simulink model "digital_filter"  (R2018b)
settings: Solver=ode4  StartTime=0.0  StopTime=0.08  FixedStep=5e-6  RelTol=1e-3
undefined symbols (not defined in the file or in its folder): DiscIntNeverNeededParam
libraries: powerlib_meascontrol x8, dsparch4 x1
settings Model: Creator=Alexey  LastModifiedBy=Alexey

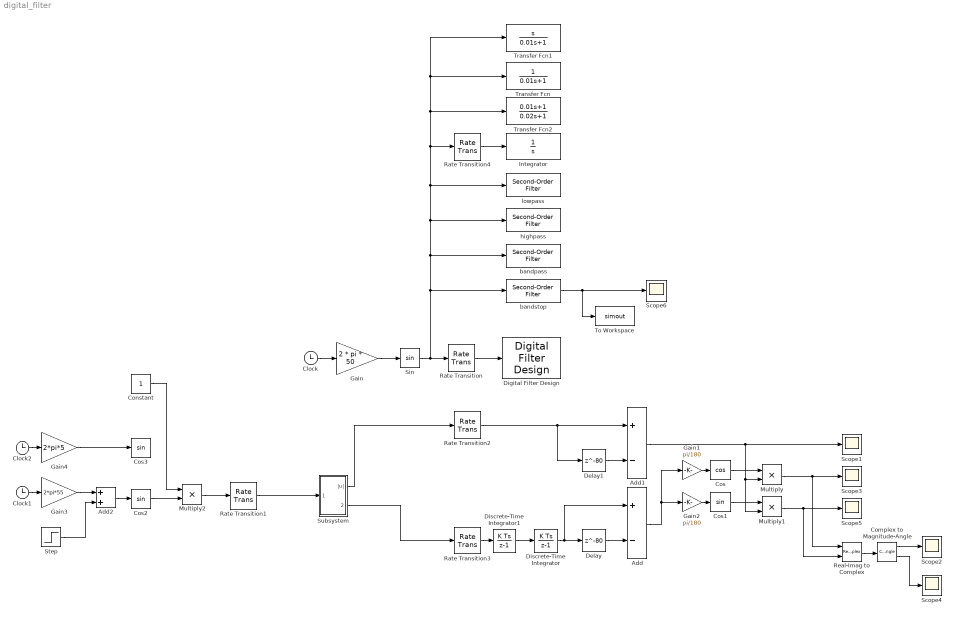
== system digital_filter ==
  Add : Sum  Inputs=+-
  Add1 : Sum  Inputs=+-
  Add2 : Sum
  Clock : Clock
  Clock1 : Clock
  Clock2 : Clock
  Complex to Magnitude-Angle : ComplexToMagnitudeAngle
  Constant : Constant
  Cos : Trigonometry  Operator=cos
  Cos1 : Trigonometry
  Cos2 : Trigonometry
  Cos3 : Trigonometry
  Delay : Delay  DelayLength=80
  Delay1 : Delay  DelayLength=80
  Digital Filter Design : dsparch4/Digital Filter Design  mwdsp_browser_bugfix_var=off
  Discrete-Time Integrator : DiscreteIntegrator  SampleTime=-1  ICPrevOutput=DiscIntNeverNeededParam  ICPrevScaledInput=DiscIntNeverNeededParam
  Discrete-Time Integrator1 : DiscreteIntegrator  SampleTime=-1  ICPrevOutput=DiscIntNeverNeededParam  ICPrevScaledInput=DiscIntNeverNeededParam
  Gain : Gain  Gain=2 * pi * 50
  Gain1 : Gain  Gain=pi/180
  Gain2 : Gain  Gain=pi/180
  Gain3 : Gain  Gain=2*pi*55
  Gain4 : Gain  Gain=2*pi*5
  Integrator : Integrator
  Multiply : Product
  Multiply1 : Product
  Multiply2 : Product
  Rate Transition : RateTransition  Integrity=off  Deterministic=off  OutPortSampleTime=1 / 4000
  Rate Transition1 : RateTransition  Integrity=off  Deterministic=off  OutPortSampleTime=1/4000
  Rate Transition2 : RateTransition  Integrity=off  Deterministic=off  OutPortSampleTime=1/4000
  Rate Transition3 : RateTransition  Integrity=off  Deterministic=off  OutPortSampleTime=1/4000
  Rate Transition4 : RateTransition  Integrity=off  Deterministic=off  OutPortSampleTime=1 / 4000
  Real-Imag to Complex : RealImagToComplex
  Scope{1..6} (6 alike) : Scope
  Sin : Trigonometry
  Step : Step  Time=0.5  After=30*pi/180  SampleTime=0
  Subsystem : Subsystem
  To Workspace : ToWorkspace  VariableName=simout  SampleTime=1/4000
  Transfer Fcn : TransferFcn  Numerator=[0 1]  Denominator=[0.01 1]
  Transfer Fcn1 : TransferFcn  Numerator=[1 0]  Denominator=[0.01 1]
  Transfer Fcn2 : TransferFcn  Numerator=[0.01 1]  Denominator=[0.02 1]
  bandpass : powerlib_meascontrol/Filters/Second-Order Filter  FilterType=Bandpass  Fo=120  Zeta=0.707  Ts=0  Initialize=off  Vac_Init="[0,  0,  60]"  Vdc_Init=0  PlotResponse=off  FreqRange=[0, 500, 1]
      settings: SourceProductName=Simscape Power Systems  SourceProductBaseCode=PS
  bandstop : powerlib_meascontrol/Filters/Second-Order Filter  FilterType=Bandstop (Notch)  Fo=120  Zeta=0.707  Ts=0  Initialize=off  Vac_Init="[0,  0,  60]"  Vdc_Init=0  PlotResponse=off  FreqRange=[0, 500, 1]
      settings: SourceProductName=Simscape Power Systems  SourceProductBaseCode=PS
  highpass : powerlib_meascontrol/Filters/Second-Order Filter  FilterType=Highpass  Fo=120  Zeta=0.707  Ts=0  Initialize=off  Vac_Init="[0,  0,  60]"  Vdc_Init=0  PlotResponse=off  FreqRange=[0, 500, 1]
      settings: SourceProductName=Simscape Power Systems  SourceProductBaseCode=PS
  lowpass : powerlib_meascontrol/Filters/Second-Order Filter  FilterType=Lowpass  Fo=120  Zeta=0.707  Ts=0  Initialize=off  Vac_Init="[0,  0,  60]"  Vdc_Init=0  PlotResponse=off  FreqRange=[0, 500, 1]
      settings: SourceProductName=Simscape Power Systems  SourceProductBaseCode=PS
  wires:
  Clock/1 -> Gain/1
  Gain/1 -> Sin/1
  Sin/1 -> bandstop/1, bandpass/1, lowpass/1, Transfer Fcn2/1, Transfer Fcn1/1, Transfer Fcn/1, Rate Transition4/1, highpass/1, Rate Transition/1
  Rate Transition/1 -> Digital Filter Design/1
  Subsystem/2(arg) -> Rate Transition3/1
  Discrete-Time Integrator/1 -> Add/1, Delay/1
  Delay/1 -> Add/2
  Add/1 -> Gain1/1, Gain2/1
  Delay1/1 -> Add1/2
  Discrete-Time Integrator1/1 -> Discrete-Time Integrator/1
  Rate Transition1/1 -> Subsystem/1(input)
  Subsystem/1(|u|) -> Rate Transition2/1
  Add1/1 -> Multiply1/2, Multiply/2, Scope1/1
  Gain1/1 -> Cos/1
  Gain2/1 -> Cos1/1
  Cos/1 -> Multiply/1
  Cos1/1 -> Multiply1/1
  Multiply/1 -> Real-Imag to Complex/1, Scope3/1
  Multiply1/1 -> Real-Imag to Complex/2, Scope5/1
  Rate Transition2/1 -> Delay1/1, Add1/1
  Rate Transition3/1 -> Discrete-Time Integrator1/1
  Clock1/1 -> Gain3/1
  Gain3/1 -> Add2/1
  Step/1 -> Add2/2
  Add2/1 -> Cos2/1
  Cos2/1 -> Multiply2/2
  Real-Imag to Complex/1 -> Complex to Magnitude-Angle/1
  Complex to Magnitude-Angle/1 -> Scope2/1
  Multiply2/1 -> Rate Transition1/1
  Clock2/1 -> Gain4/1
  Gain4/1 -> Cos3/1
  Complex to Magnitude-Angle/2 -> Scope4/1
  Constant/1 -> Multiply2/1
  bandstop/1 -> To Workspace/1, Scope6/1
  Rate Transition4/1 -> Integrator/1

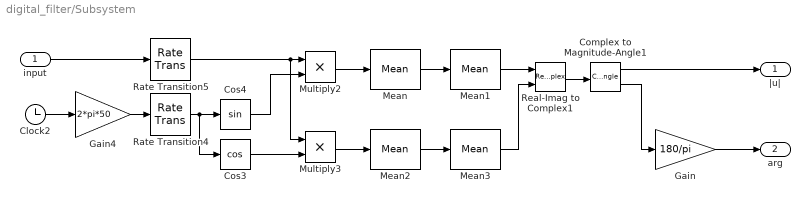
== system digital_filter/Subsystem ==
  input : Inport
  Clock2 : Clock
  Complex to Magnitude-Angle1 : ComplexToMagnitudeAngle
  Cos3 : Trigonometry  Operator=cos
  Cos4 : Trigonometry
  Gain : Gain  Gain=180/pi
  Gain4 : Gain  Gain=2*pi*50
  Mean{,1..3} (4 alike) : powerlib_meascontrol/Measurements/Mean  Freq=50  Vinit=0  Ts=1/4000
  Multiply2 : Product
  Multiply3 : Product
  Rate Transition4 : RateTransition  Integrity=off  Deterministic=off  OutPortSampleTime=1/4000
  Rate Transition5 : RateTransition  Integrity=off  Deterministic=off  OutPortSampleTime=1/4000
  Real-Imag to Complex1 : RealImagToComplex
  |u| : Outport
  arg : Outport  Port=2
  wires:
  Real-Imag to Complex1/1 -> Complex to Magnitude-Angle1/1
  Rate Transition4/1 -> Cos3/1, Cos4/1
  Clock2/1 -> Gain4/1
  Cos3/1 -> Multiply3/2
  Rate Transition5/1 -> Multiply3/1, Multiply2/1
  Multiply2/1 -> Mean/1
  Mean1/1 -> Real-Imag to Complex1/1
  Mean/1 -> Mean1/1
  Gain4/1 -> Rate Transition4/1
  Multiply3/1 -> Mean2/1
  Mean2/1 -> Mean3/1
  Cos4/1 -> Multiply2/2
  Mean3/1 -> Real-Imag to Complex1/2
  Complex to Magnitude-Angle1/1 -> |u|/1
  Complex to Magnitude-Angle1/2 -> Gain/1
  input/1 -> Rate Transition5/1
  Gain/1 -> arg/1
